simulink model "HW2_es3"  (R2024a)
settings: Solver=VariableStepAuto  StartTime=0.0  StopTime=2*pi  RelTol=1e-3
values from neighbouring files (symbols this model uses):
  a = load('ERROR_NORM_0.01.mat')    [H2.m]    (also in H2_es3.m = 1; H2_es4.m = 1)
  r = 1    [H2_es3.m]
  w_rand = rand(1,1)*pi*2    [H2_es3.m]
libraries: robotmobilelib x2
settings Model: Creator=Strix  LastModifiedBy=Strix

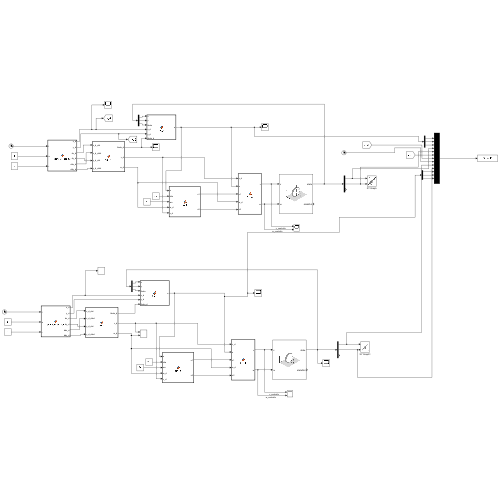
[thumbnail: Simulink's stored preview of the top-level diagram]
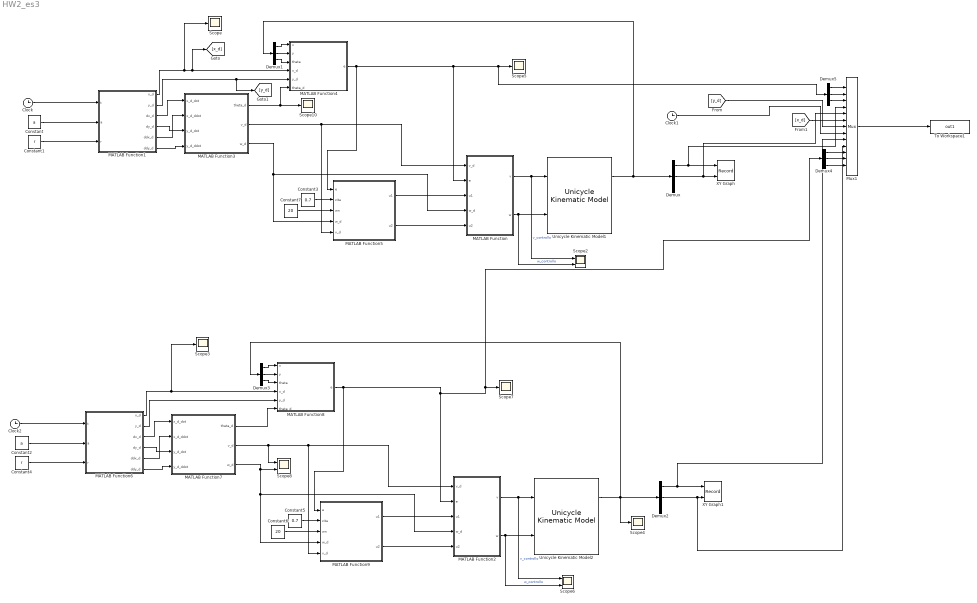
== system HW2_es3 ==
  Clock : Clock
  Clock1 : Clock
  Clock2 : Clock
  Constant : Constant  Value=a
  Constant1 : Constant  Value=r
  Constant2 : Constant  Value=a
  Constant3 : Constant  Value=0.7
  Constant4 : Constant  Value=r
  Constant5 : Constant  Value=0.7
  Constant6 : Constant  Value=20
  Constant7 : Constant  Value=20
  Demux{,1..5} (6 alike) : Demux  Outputs=3
  MATLAB Function : MATLAB Function  TreatAsAtomicUnit=on
  MATLAB Function1 : MATLAB Function  TreatAsAtomicUnit=on
  MATLAB Function2 : MATLAB Function  TreatAsAtomicUnit=on
  MATLAB Function3 : MATLAB Function  TreatAsAtomicUnit=on
  MATLAB Function4 : MATLAB Function  TreatAsAtomicUnit=on
  MATLAB Function5 : MATLAB Function  TreatAsAtomicUnit=on
  MATLAB Function6 : MATLAB Function  TreatAsAtomicUnit=on
  MATLAB Function7 : MATLAB Function  TreatAsAtomicUnit=on
  MATLAB Function8 : MATLAB Function  TreatAsAtomicUnit=on
  MATLAB Function9 : MATLAB Function  TreatAsAtomicUnit=on
  Mux1 : Mux  Inputs=13
  Scope{,3..5,7,10} (6 alike) : Scope
  Scope2 : Scope  NumInputPorts=2
  Scope6 : Scope  NumInputPorts=2
  Scope8 : Scope  NumInputPorts=2
  To Workspace1 : ToWorkspace  VariableName=out1  SampleTime=-1
  Unicycle Kinematic Model1 : robotmobilelib/Unicycle Kinematic Model  VehicleInputs=Vehicle Speed & Heading Angular Velocity  WheelRadius=0.1  WheelSpeedRange=[-Inf Inf]  InitialState=[r+0.5*cos(w_rand);0.5*sin(w_rand); 0]  SimulateUsing=Interpreted execution
  Unicycle Kinematic Model2 : robotmobilelib/Unicycle Kinematic Model  VehicleInputs=Vehicle Speed & Heading Angular Velocity  WheelRadius=0.1  WheelSpeedRange=[-Inf Inf]  InitialState=[r+0.5*cos(w_rand);0.5*sin(w_rand); 0]  SimulateUsing=Interpreted execution
  XY Graph : Record  FileSettingsInternal="{\"entries\":[{\"content\":{\"excelSettings\":{\"content\":{},\"type\":\"Streamout.ExcelSettings\"}},\"type\":\"Streamout.FileSettingStorage\",\"uuid\":\"\"}],\"packageUris\":[\"http:\\/\\/schema.mathworks.com\\/mf0\\/streamout_blocks\\/R2020a\"],\"version\":\"1.0\"}"  Layout=[1 1]  SignalsInternal="{\"entries\":[{\"content\":{\"signals\":[{\"content\":{\"blockPath\":[],\"dimensions\":[1],\"domain\":\"\",\"lineColor\":\"#0072bd\",\"lineWidth\":2,\"port\":1,\"sid\":[\"\"],\"signalID\":1,\"signalName\":\"Demux:1\"},\"type\":\"RecordBlkView.Signal\",\"uuid\":\"\"},{\"content\":{\"blockPath\":[],\"dimensions\":[1],\"domain\":\"\",\"lineColor\":\"#d95319\",\"lineWidth\":2,\"port\":2,\"sid\":[\"\"],\"signalID\":2,\"signalName\":\"Demux:2\"},\"type\":\"RecordBlkView.Signal\",\"uuid\":\"\"}]},\"type\":\"RecordBlkView.InputSignals\",\"uuid\":\"\"}],\"packageUris\":[\"http:\\/\\/schema.mathworks.com\\/mf0\\/streamout_blocks\\/R2020a\"],\"version\":\"1.0\"}"  VisualizationBindings="{\"xyplotplugin\":{\"info\":[{\"series\":[],\"subplotID\":1}]}}"  CompatibilityTag=XY
  XY Graph1 : Record  FileSettingsInternal="{\"entries\":[{\"content\":{\"excelSettings\":{\"content\":{},\"type\":\"Streamout.ExcelSettings\"}},\"type\":\"Streamout.FileSettingStorage\",\"uuid\":\"\"}],\"packageUris\":[\"http:\\/\\/schema.mathworks.com\\/mf0\\/streamout_blocks\\/R2020a\"],\"version\":\"1.0\"}"  Layout=[1 1]  SignalsInternal="{\"entries\":[{\"content\":{\"signals\":[{\"content\":{\"blockPath\":[],\"dimensions\":[1],\"domain\":\"\",\"lineColor\":\"#a2142f\",\"plots\":[ 1 ],\"port\":1,\"sid\":[\"\"],\"signalID\":1,\"signalName\":\"Demux2:1\"},\"type\":\"RecordBlkView.Signal\",\"uuid\":\"\"},{\"content\":{\"blockPath\":[],\"dimensions\":[1],\"domain\":\"\",\"lineColor\":\"#139fff\",\"plots\":[ 1 ],\"port\":2,\"sid\":[\"\"],\"signalID\":2,\"signalName\":\"Demux2:2\"},\"type\":\"RecordBlkView.Signal\",\"uuid\":\"\"}]},\"type\":\"RecordBlkView.InputSignals\",\"uuid\":\"\"}],\"packageUris\":[\"http:\\/\\/schema.mathworks.com\\/mf0\\/streamout_blocks\\/R2020a\"],\"version\":\"1.0\"}"  VisualizationBindings="{\"xyplotplugin\":{\"info\":[{\"series\":[{\"bindingParametersList\":[{\"parameter\":\"X-Axis\",\"signalID\":1,\"signalName\":\"Demux2:1\"},{\"parameter\":\"Y-Axis\",\"signalID\":2,\"signalName\":\"Demux2:2\"}],\"seriesID\":0}],\"subplotID\":1}]}}"  CompatibilityTag=XY
  wires:
  Mux1/1 -> To Workspace1/1
  MATLAB Function/2(w) -> Scope2/2, Unicycle Kinematic Model1/2  "w_controllo"
  MATLAB Function/1(v) -> Scope2/1, Unicycle Kinematic Model1/1  "v_controllo"
  Demux/2 -> XY Graph/2, Mux1/5
  Demux/1 -> XY Graph/1, Mux1/4
  Constant1/1 -> MATLAB Function1/3(r)
  Constant/1 -> MATLAB Function1/2(a)
  Clock/1 -> MATLAB Function1/1(t)
  MATLAB Function1/1(x_d) -> Scope/1, [x_d], MATLAB Function4/4(x_d)
  MATLAB Function1/2(y_d) -> [y_d], MATLAB Function4/5(y_d)
  MATLAB Function3/2(v_d) -> MATLAB Function/1(v_d), MATLAB Function5/5(v_d)
  MATLAB Function3/3(w_d) -> MATLAB Function5/4(w_d), MATLAB Function/4(w_d)
  MATLAB Function3/1(theta_d) -> Scope10/1, MATLAB Function4/6(theta_d)
  Unicycle Kinematic Model1/1 -> Demux/1, Demux1/1
  Demux1/3 -> MATLAB Function4/3(theta)
  Demux1/2 -> MATLAB Function4/2(y)
  Demux1/1 -> MATLAB Function4/1(x)
  MATLAB Function5/1(u1) -> MATLAB Function/3(u1)
  MATLAB Function5/2(u2) -> MATLAB Function/5(u2)
  Constant3/1 -> MATLAB Function5/2(zita)
  Constant7/1 -> MATLAB Function5/3(wn)
  MATLAB Function4/1(e) -> MATLAB Function/2(e), Demux5/1, Scope5/1, MATLAB Function5/1(e)
  MATLAB Function1/3(dx_d) -> MATLAB Function3/1(x_d_dot)
  MATLAB Function1/4(dy_d) -> MATLAB Function3/3(y_d_dot)
  MATLAB Function1/5(ddx_d) -> MATLAB Function3/2(x_d_ddot)
  MATLAB Function1/6(ddy_d) -> MATLAB Function3/4(y_d_ddot)
  Demux5/1 -> Mux1/1
  Demux5/2 -> Mux1/2
  Demux5/3 -> Mux1/3
  [x_d] -> Mux1/6
  [y_d] -> Mux1/7
  Clock1/1 -> Mux1/8
  Demux3/3 -> MATLAB Function8/3(theta)
  MATLAB Function6/1(x_d) -> Scope3/1, MATLAB Function8/4(x_d)
  MATLAB Function6/6(ddy_d) -> MATLAB Function7/4(y_d_ddot)
  MATLAB Function6/5(ddx_d) -> MATLAB Function7/2(x_d_ddot)
  Demux3/1 -> MATLAB Function8/1(x)
  Demux3/2 -> MATLAB Function8/2(y)
  MATLAB Function6/4(dy_d) -> MATLAB Function7/3(y_d_dot)
  MATLAB Function9/2(u2) -> MATLAB Function2/5(u2)
  MATLAB Function7/1(theta_d) -> MATLAB Function8/6(theta_d)
  Constant5/1 -> MATLAB Function9/2(zita)
  Demux2/1 -> Mux1/9, XY Graph1/1
  MATLAB Function7/2(v_d) -> Scope8/1, MATLAB Function2/1(v_d), MATLAB Function9/5(v_d)
  Unicycle Kinematic Model2/1 -> Scope4/1, Demux2/1, Demux3/1
  MATLAB Function9/1(u1) -> MATLAB Function2/3(u1)
  Constant6/1 -> MATLAB Function9/3(wn)
  MATLAB Function6/2(y_d) -> MATLAB Function8/5(y_d)
  Constant4/1 -> MATLAB Function6/3(r)
  Clock2/1 -> MATLAB Function6/1(t)
  Constant2/1 -> MATLAB Function6/2(a)
  MATLAB Function2/2(w) -> Scope6/2, Unicycle Kinematic Model2/2  "w_controllo"
  MATLAB Function8/1(e) -> MATLAB Function2/2(e), Demux4/1, Scope7/1, MATLAB Function9/1(e)
  Demux2/2 -> XY Graph1/2, Mux1/10
  MATLAB Function2/1(v) -> Scope6/1, Unicycle Kinematic Model2/1  "v_controllo"
  MATLAB Function6/3(dx_d) -> MATLAB Function7/1(x_d_dot)
  MATLAB Function7/3(w_d) -> MATLAB Function9/4(w_d), MATLAB Function2/4(w_d), Scope8/2
  Demux4/1 -> Mux1/11
  Demux4/2 -> Mux1/12
  Demux4/3 -> Mux1/13

== matlab function HW2_es3/MATLAB Function7 ==
  data: x_d_dot input; theta_d output; v_d output; w_d output; x_d_ddot input; y_d_dot input; y_d_ddot input
function [theta_d,v_d,w_d] = fcn_1(x_d_dot,x_d_ddot,y_d_dot,y_d_ddot)

    theta_d = atan2(y_d_dot, x_d_dot);
    v_d = sqrt(x_d_dot^2 + y_d_dot^2);
    w_d = (y_d_ddot* x_d_dot - x_d_ddot .* y_d_dot) ./ ((x_d_dot).^2 + (y_d_dot).^2);

== matlab function HW2_es3/MATLAB Function8 ==
  data: x input; e output; y input; theta input; x_d input; y_d input; theta_d input
function e = fcn_2(x,y,theta,x_d,y_d,theta_d)

T=[cos(theta) sin(theta) 0
   -sin(theta) cos(theta) 0
    0 0 1];

q=[x,y,theta];
q_d=[x_d,y_d,theta_d];


e=T*(q_d-q)';

== matlab function HW2_es3/MATLAB Function9 ==
  data: e input; u1 output; zita input; wn input; w_d input; v_d input; u2 output
function [u1,u2] = fcn_3(e,zita,wn,w_d,v_d)


k1=2*zita*wn;
k2=(wn^2);
k3=2*zita*wn;

u1=-k1*e(1);
u2=-k2*v_d*sin(e(3))*e(2)/e(3)-k3*e(3);

== matlab function HW2_es3/MATLAB Function1 ==
  data: t input; x_d output; a input; r input; y_d output; dx_d output; dy_d output; ddx_d output; ddy_d output
function [x_d, y_d, dx_d, dy_d, ddx_d, ddy_d] = bernoulli_traj_full(t, a, r)
% Traiettoria lemniscata di Bernoulli con derivate prima e seconda


if t>4*pi/(a+1)
t=4*pi/(a+1);
end

omega = a + 1;
s = sin(omega * t);
c = cos(omega * t);
D = 1 + s^2;
D2 = D^2;
D3 = D^3;

% Posizione
x_d = r * c / D;
y_d = r * c * s / D;

% Derivate prime
num_dx = -omega * s * D + (-omega * c) * (2 * s * c);
dx_d = r * num_dx / D2;

num_dy = omega * (c^2 - s^2) * D - omega * 2 * s^2 * c^2;
dy_d = r * num_dy / D2;

% Derivate seconde
% Seconda derivata di x_d
ds = omega * c;
dc = -omega * s;
dD = 2 * s * ds; % = 2*omega*s*cos(omega*t)
ddc = -omega^2 * c;
dds = -omega^2 * s;
ddD = 2 * (ds^2 + s * dds);

num_ddx = ddc * D - 2 * dc * dD - c * ddD;
ddx_d = r * num_ddx / D2 + r * 2 * c * dD^2 / D3;

% Seconda derivata di y_d
% y = r * c * s / D
dcs = dc * s + c * ds;
ddcs = ddc * s + 2 * dc * ds + c * dds;

num_ddy = ddcs * D - 2 * dcs * dD - c * s * ddD;
ddy_d = r * num_ddy / D2 + r * 2 * c * s * dD^2 / D3;



ddy_d=(4*r*omega^2 *(7 + 3*cos(2*t*omega))*sin(2*t*omega))/(-3 + cos(2*t*omega))^3;

end

== matlab function HW2_es3/MATLAB Function ==
  data: v_d input; v output; e input; w output; u1 input; w_d input; u2 input
function [v,w] = fcn_4(v_d,e,u1,w_d,u2)

v=v_d*cos(e(3))-u1;
w=w_d-u2;

== matlab function HW2_es3/MATLAB Function2 ==
  data: v_d input; v output; e input; w output; u1 input; w_d input; u2 input
function [v,w] = fcn_4(v_d,e,u1,w_d,u2)

v=v_d*cos(e(3))-u1;
w=w_d-u2;

== matlab function HW2_es3/MATLAB Function3 ==
  data: x_d_dot input; theta_d output; v_d output; w_d output; x_d_ddot input; y_d_dot input; y_d_ddot input
function [theta_d,v_d,w_d] = fcn_1(x_d_dot,x_d_ddot,y_d_dot,y_d_ddot)

    theta_d = atan2(y_d_dot, x_d_dot);
    v_d = sqrt(x_d_dot^2 + y_d_dot^2);
    w_d = (y_d_ddot* x_d_dot - x_d_ddot .* y_d_dot) ./ ((x_d_dot).^2 + (y_d_dot).^2);

== matlab function HW2_es3/MATLAB Function4 ==
  data: x input; e output; y input; theta input; x_d input; y_d input; theta_d input
function e = fcn_2(x,y,theta,x_d,y_d,theta_d)

T=[cos(theta) sin(theta) 0
   -sin(theta) cos(theta) 0
    0 0 1];

q=[x,y,theta];
q_d=[x_d,y_d,theta_d];


e=T*(q_d-q)';

== matlab function HW2_es3/MATLAB Function5 ==
  data: e input; u1 output; zita input; wn input; w_d input; v_d input; u2 output
function [u1,u2] = fcn_3(e,zita,wn,w_d,v_d)


k1=2*zita*wn;
k2=(wn^2-w_d)/v_d;
k3=2*zita*wn;

u1=-k1*e(1);
u2=-k2*e(2)-k3*e(3);

== matlab function HW2_es3/MATLAB Function6 ==
  data: t input; x_d output; a input; r input; y_d output; dx_d output; dy_d output; ddx_d output; ddy_d output
function [x_d, y_d, dx_d, dy_d, ddx_d, ddy_d] = bernoulli_traj_full(t, a, r)
% Traiettoria lemniscata di Bernoulli con derivate prima e seconda


if t>4*pi/(a+1)
t=4*pi/(a+1);
end

omega = a + 1;
s = sin(omega * t);
c = cos(omega * t);
D = 1 + s^2;
D2 = D^2;
D3 = D^3;

% Posizione
x_d = r * c / D;
y_d = r * c * s / D;

% Derivate prime
num_dx = -omega * s * D + (-omega * c) * (2 * s * c);
dx_d = r * num_dx / D2;

num_dy = omega * (c^2 - s^2) * D - omega * 2 * s^2 * c^2;
dy_d = r * num_dy / D2;

% Derivate seconde
% Seconda derivata di x_d
ds = omega * c;
dc = -omega * s;
dD = 2 * s * ds; % = 2*omega*s*cos(omega*t)
ddc = -omega^2 * c;
dds = -omega^2 * s;
ddD = 2 * (ds^2 + s * dds);

num_ddx = ddc * D - 2 * dc * dD - c * ddD;
ddx_d = r * num_ddx / D2 + r * 2 * c * dD^2 / D3;

% Seconda derivata di y_d
% y = r * c * s / D
dcs = dc * s + c * ds;
ddcs = ddc * s + 2 * dc * ds + c * dds;

num_ddy = ddcs * D - 2 * dcs * dD - c * s * ddD;
ddy_d = r * num_ddy / D2 + r * 2 * c * s * dD^2 / D3;



ddy_d=(4*r*omega^2 *(7 + 3*cos(2*t*omega))*sin(2*t*omega))/(-3 + cos(2*t*omega))^3;



% if t>4*pi/(a+1)
% dx_d=0; dy_d=0; ddx_d=0; ddy_d=0;
% end

end
